simulink model "Missile_Guidance_Solution"  (R2023b)
settings: Solver=ode45  StartTime=0.0  StopTime=20  RelTol=1e-3  AbsTol=1e-6
PreLoadFcn:
  | aero_guid_dat
StopFcn:
  | aero_guid_plot
undefined symbols (not defined in the file or in its folder): Beamwidth, Cm_el, Cm_q, Cz_el, d2r, d_ref, fin_max, fin_min, g, h_ini, K_r, Ks, l_acc, max_acc, max_gimbal, min_gimbal, pos_tgt, S_ref, theta_tgt, Thrust, tors, v_tgt, wgyro, wn_hom, x_ini
libraries: simulink_need_slupdate x11, aerospace x4, aerolibanim x1, simulink x1
CloseFcn:
  | h=findobj('type','figure');if ~isempty(h);close(h);end
Description:
  | Dynamics of a missile engaging a target which is flying straight and level
settings Model: PauseTimes=6  Creator=The MathWorks, Inc.  LastModifiedBy=AmitW
settings SolverCC: AutoScaleAbsTol=off  AlgebraicLoopSolver=TrustRegion
settings DataIOCC: SaveFormat=Array  SaveOutput=off  ReturnWorkspaceOutputs=off  StateSaveName=xbase  OutputSaveName=ybase  SignalLoggingName=sigsOut
settings OptimizationCC: BlockReduction=off  ReuseModelBlockBuffer=off  ExpressionDepthLimit=2147483647  InitFltsAndDblsToZero=on  LifeSpan=inf
settings DebuggingCC: SaveWithParameterizedLinksMsg=none  SignalResolutionControl=TryResolveAllWithWarning  MultiTaskDSMMsg=warning  MultiTaskCondExecSysMsg=none  SigSpecEnsureSampleTimeMsg=none  FcnCallInpInsideContextMsg=warning  UnconnectedInputMsg=warning  UnconnectedOutputMsg=warning  UnconnectedLineMsg=warning  StateNameClashWarn=warning  SFUnexpectedBacktrackingDiag=warning  SFNoUnconditionalDefaultTransitionDiag=warning  SFExecutionAtInitializationDiag=none  ArithmeticOperatorsInVariantConditions=warning
settings HardwareCC: ProdBitPerPointer=32  ProdBitPerSizeT=32  ProdBitPerPtrDiffT=32  ProdLargestAtomicFloat=None  ProdIntDivRoundTo=Undefined  ProdEndianess=Unspecified  ProdWordSize=32  ProdHWDeviceType=32-bit Generic
settings ModelReferenceCC: EnableRefExpFcnMdlSchedulingChecks=on  PropagateSignalLabelsOutOfModel=off
settings SFSimCC: SimUseLocalCustomCode=off  SimParseCustomCode=off  CustomCodeUndefinedFunction=UseInterfaceOnly
settings RTWCC: RTWUseLocalCustomCode=off
settings CodeAppCC: StateflowObjectComments=on
settings GRTTargetCC: TargetFcnLib=ansi_tfl_tmw.mat  TargetLangStandard=C89/C90 (ANSI)  CombineOutputUpdateFcns=off  GRTInterface=on
settings ConfigComp: CovMetricSettings=d  CovSaveCumulativeToWorkspaceVar=on  CovSaveSingleToWorkspaceVar=on  CovExternalEMLEnable=off  CovSFcnEnable=off

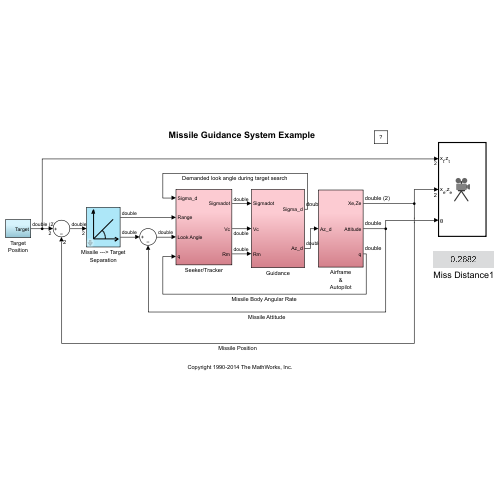
[thumbnail: Simulink's stored preview of the top-level diagram]
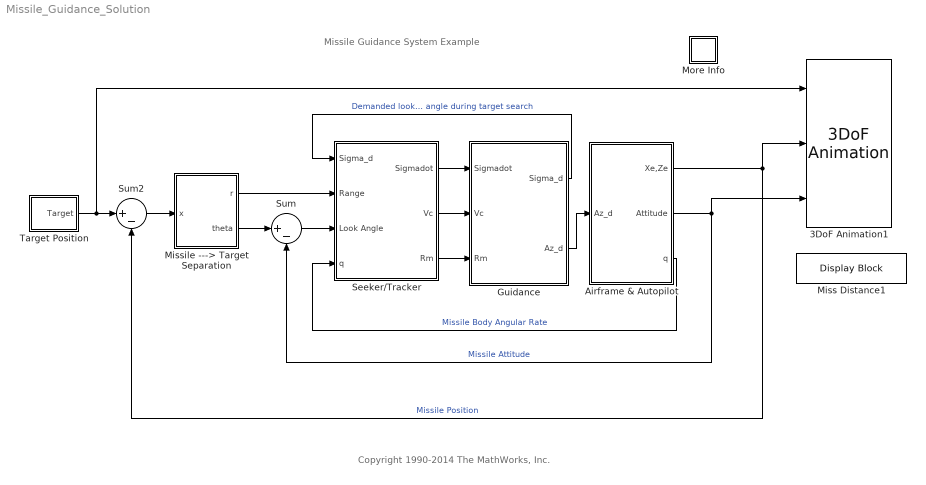
== system Missile_Guidance_Solution ==
  note: Copyright 1990-2014 The MathWorks, Inc.
  note: Missile Guidance System Example
  3DoF Animation1 : aerolibanim/3DoF Animation  u1=[0 5000 -2000 2000 -5050 -3050]  u2=0.01  u3=2.0  u5=Fixed position  u6=[2000 500 -3150]  u7=10  u8=on
  Airframe & Autopilot : Subsystem
  Guidance : Subsystem
  Miss Distance1 : DisplayBlock  LabelPosition=Hide  Transparency=1
  Missile ---> Target Separation : Subsystem  mask(Cart2Polar){}
      mask help:
      | Transformation from cartesian to polar coordinates.
      | [x, y] -> [r, theta]
      |
      | r = sqrt(x^2 + y^2);
      | theta = atan(y/x);
      mask Help: Unmask this block for more help.
      mask Display: plot(0,0,100,100,[24,20,15,20,20],[85,95,85,95,20],[80,20,95,85,95,85],[70,20,20,15,20,24],[56,56,55,52,50,46],[20,26,31,35,38,42])
  More Info : Subsystem
      settings: OpenFcn=showExample('simulink_aerospace/DesigningAGuidanceSystemInMATLABAndSimulinkExample')
      mask Display: disp('?')
  Seeker/Tracker : Subsystem
  Sum : Sum  Inputs=|+-  InputSameDT=on  SaturateOnIntegerOverflow=on  OutDataTypeStr=Inherit: Same as first input
  Sum2 : Sum  Inputs=|+-  InputSameDT=on  SaturateOnIntegerOverflow=on  OutDataTypeStr=Inherit: Same as first input
  Target Position : Subsystem
  wires:
  Missile ---> Target Separation/2(theta) -> Sum/1
  Guidance/2(Az_d) -> Airframe & Autopilot/1(Az_d)
  Seeker/Tracker/2(Vc) -> Guidance/2(Vc)
  Seeker/Tracker/3(Rm) -> Guidance/3(Rm)
  Seeker/Tracker/1(Sigmadot) -> Guidance/1(Sigmadot)
  Sum/1 -> Seeker/Tracker/3(Look Angle)
  Airframe & Autopilot/3(q) -> Seeker/Tracker/4(q)  "Missile Body Angular Rate"
  Guidance/1(Sigma_d) -> Seeker/Tracker/1(Sigma_d)  "Demanded look angle during target search"
  Missile ---> Target Separation/1(r) -> Seeker/Tracker/2(Range)
  Airframe & Autopilot/1(Xe,Ze) -> 3DoF Animation1/2, Sum2/2  "Missile Position"
  Airframe & Autopilot/2(Attitude) -> 3DoF Animation1/3, Sum/2  "Missile Attitude"
  Target Position/1(Target) -> 3DoF Animation1/1, Sum2/1
  Sum2/1 -> Missile ---> Target Separation/1(x)

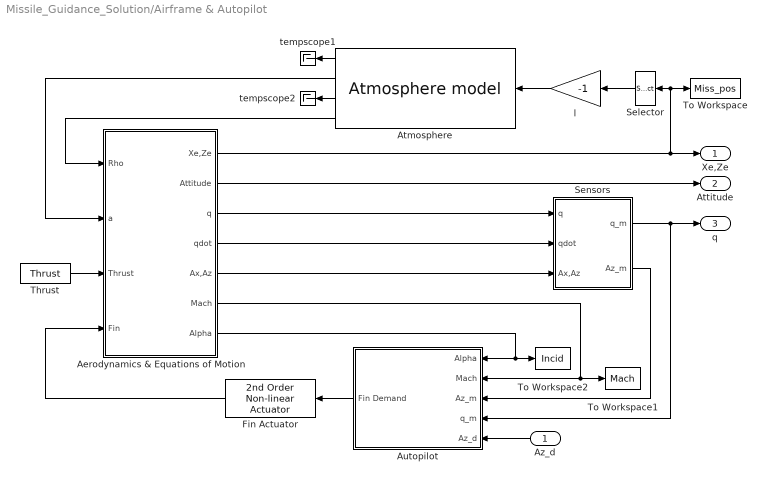
== system Missile_Guidance_Solution/Airframe & Autopilot ==
  Az_d : Inport
  Aerodynamics & Equations of Motion : Subsystem
  Atmosphere : aerospace/Atmosphere/Atmosphere model
  Autopilot : Subsystem
  Fin Actuator : aerospace/Actuators/2nd Order Non-linear Actuator  wn_fin=wn_fin  z_fin=z_fin  fin_max=fin_max  fin_min=fin_min  fin_maxrate=fin_maxrate  fin_act_0=fin_act_0
  Selector : Selector  InputPortWidth=2  IndexOptions=Index vector (dialog)  Indices=[2]  OutputSizes=1
  Sensors : Subsystem
  Thrust : Constant  Value=Thrust
  To Workspace : ToWorkspace  VariableName=Miss_pos  SaveFormat=Structure With Time  SampleTime=-1
  To Workspace1 : ToWorkspace  VariableName=Mach  SaveFormat=Structure With Time  SampleTime=-1
  To Workspace2 : ToWorkspace  VariableName=Incid  SaveFormat=Structure With Time  SampleTime=-1
  l : Gain  Gain=-1  SaturateOnIntegerOverflow=on  OutDataTypeStr=Inherit: Same as input  ParamDataTypeStr=Inherit: Same as input
  tempscope1 : Terminator
  tempscope2 : Terminator
  Xe,Ze : Outport  InitialOutput=0  VectorParamsAs1DForOutWhenUnconnected=off
  Attitude : Outport  Port=2  InitialOutput=0  VectorParamsAs1DForOutWhenUnconnected=off
  q : Outport  Port=3  InitialOutput=0  VectorParamsAs1DForOutWhenUnconnected=off
  wires:
  Aerodynamics & Equations of Motion/2(Attitude) -> Attitude/1
  Thrust/1 -> Aerodynamics & Equations of Motion/3(Thrust)
  Atmosphere/3 -> tempscope2/1
  Atmosphere/4 -> Aerodynamics & Equations of Motion/1(Rho)
  Atmosphere/1 -> tempscope1/1
  Atmosphere/2 -> Aerodynamics & Equations of Motion/2(a)
  Selector/1 -> l/1
  l/1 -> Atmosphere/1
  Aerodynamics & Equations of Motion/5(Ax,Az) -> Sensors/3(Ax,Az)
  Aerodynamics & Equations of Motion/4(qdot) -> Sensors/2(qdot)
  Aerodynamics & Equations of Motion/1(Xe,Ze) -> Xe,Ze/1, To Workspace/1, Selector/1
  Az_d/1 -> Autopilot/5(Az_d)
  Autopilot/1(Fin Demand) -> Fin Actuator/1
  Fin Actuator/1 -> Aerodynamics & Equations of Motion/4(Fin)
  Aerodynamics & Equations of Motion/7(Alpha) -> Autopilot/1(Alpha), To Workspace2/1
  Sensors/2(Az_m) -> Autopilot/3(Az_m)
  Aerodynamics & Equations of Motion/6(Mach) -> Autopilot/2(Mach), To Workspace1/1
  Sensors/1(q_m) -> Autopilot/4(q_m), q/1
  Aerodynamics & Equations of Motion/3(q) -> Sensors/1(q)

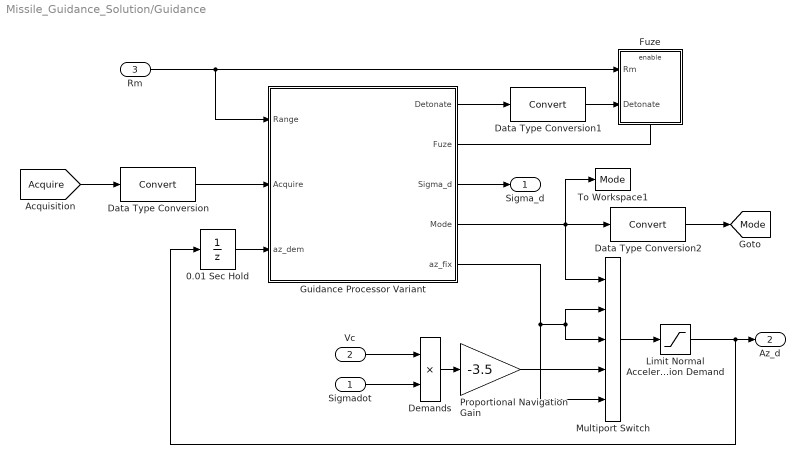
== system Missile_Guidance_Solution/Guidance ==
  Sigmadot : Inport
  Vc : Inport  Port=2
  Rm : Inport  Port=3
  0.01 Sec Hold : UnitDelay  SampleTime=0.01  HasFrameUpgradeWarning=on
  Data Type Conversion : DataTypeConversion  SaturateOnIntegerOverflow=off  RndMeth=Floor
  Data Type Conversion1 : DataTypeConversion  SaturateOnIntegerOverflow=off  RndMeth=Floor
  Data Type Conversion2 : DataTypeConversion  SaturateOnIntegerOverflow=off  RndMeth=Floor
  Demands : Product  InputSameDT=on  SaturateOnIntegerOverflow=on  OutDataTypeStr=Inherit: Same as first input
  Fuze : Subsystem  TreatAsAtomicUnit=on
  Guidance Processor Variant : Subsystem  Variant=on  VariantControlMode=label  LabelModeActiveChoice=Guid_Stateflow  mask(Guidance Processor){VarModel=Stateflow}
      mask prompts: VarModel "Guidance logic implementation"
      mask help:
      | Guidance missile logic.
      | The process works at 100 Hertz.
      mask init:
      | set_param(gcb, 'OverrideUsingVariant', ['Guid_' VarModel]);
      mask TypeOptions VarModel: Matlab | Stateflow
  "Limit Normal Acceleration Demand " : Saturate  UpperLimit=max_acc  LowerLimit=-max_acc
  Multiport Switch : MultiPortSwitch  Inputs=4
  Proportional Navigation Gain : Gain  Gain=-3.5  SaturateOnIntegerOverflow=on  OutDataTypeStr=Inherit: Same as input  ParamDataTypeStr=Inherit: Same as input
  To Workspace1 : ToWorkspace  VariableName=Mode  SaveFormat=Structure With Time
  Sigma_d : Outport  VectorParamsAs1DForOutWhenUnconnected=off
  Az_d : Outport  Port=2  VectorParamsAs1DForOutWhenUnconnected=off
  tag scope: Mode=global
  wires:
  Guidance Processor Variant/3(Sigma_d) -> Sigma_d/1
  [Acquire] -> Data Type Conversion/1
  Multiport Switch/1 -> "Limit Normal Acceleration Demand "/1
  Guidance Processor Variant/1(Detonate) -> Data Type Conversion1/1
  "Limit Normal Acceleration Demand "/1 -> Az_d/1, 0.01 Sec Hold/1
  Guidance Processor Variant/5(az_fix) -> Multiport Switch/2, Multiport Switch/3, Multiport Switch/5
  0.01 Sec Hold/1 -> Guidance Processor Variant/3(az_dem)
  Sigmadot/1 -> Demands/2
  Proportional Navigation Gain/1 -> Multiport Switch/4
  Vc/1 -> Demands/1
  Demands/1 -> Proportional Navigation Gain/1
  Rm/1 -> Guidance Processor Variant/1(Range), Fuze/1(Rm)
  Guidance Processor Variant/2(Fuze) -> Fuze/Enable
  Guidance Processor Variant/4(Mode) -> Data Type Conversion2/1, To Workspace1/1, Multiport Switch/1
  Data Type Conversion/1 -> Guidance Processor Variant/2(Acquire)
  Data Type Conversion1/1 -> Fuze/2(Detonate)
  Data Type Conversion2/1 -> [Mode]

== system Missile_Guidance_Solution/Missile ---> Target Separation ==
  x : Inport
  Range : Fcn  Expr=hypot(u[1],u[2])
  Sightline Angle : Fcn  Expr=atan2(-u[2],u[1])
  r : Outport  InitialOutput=0  VectorParamsAs1DForOutWhenUnconnected=off
  theta : Outport  Port=2  InitialOutput=0  VectorParamsAs1DForOutWhenUnconnected=off
  wires:
  x/1 -> Sightline Angle/1, Range/1
  Range/1 -> r/1
  Sightline Angle/1 -> theta/1

== system Missile_Guidance_Solution/More Info ==

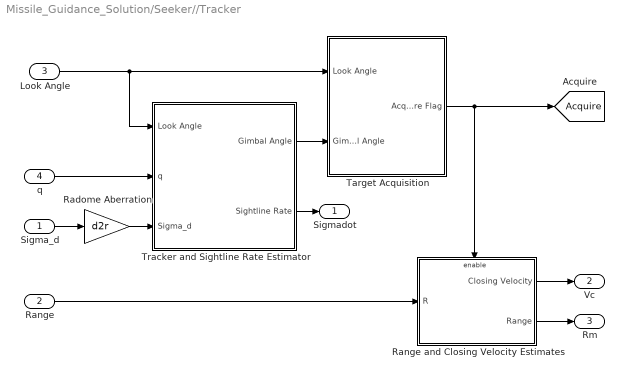
== system Missile_Guidance_Solution/Seeker//Tracker ==
  Sigma_d : Inport
  Range : Inport  Port=2
  Look Angle : Inport  Port=3
  q : Inport  Port=4
  Radome Aberration : Gain  Gain=d2r  SaturateOnIntegerOverflow=on  OutDataTypeStr=Inherit: Same as input  ParamDataTypeStr=Inherit: Same as input
  Range and Closing Velocity Estimates : Subsystem  TreatAsAtomicUnit=on
  Target Acquisition : Subsystem
  Tracker and Sightline Rate Estimator : Subsystem
  Sigmadot : Outport  VectorParamsAs1DForOutWhenUnconnected=off
  Vc : Outport  Port=2  VectorParamsAs1DForOutWhenUnconnected=off
  Rm : Outport  Port=3  VectorParamsAs1DForOutWhenUnconnected=off
  tag scope: Acquire=global
  wires:
  Tracker and Sightline Rate Estimator/2(Sightline Rate) -> Sigmadot/1
  Radome Aberration/1 -> Tracker and Sightline Rate Estimator/3(Sigma_d)
  Tracker and Sightline Rate Estimator/1("Gimbal Angle ") -> Target Acquisition/2(Gimbal Angle)
  Target Acquisition/1(Acquire Flag) -> [Acquire], Range and Closing Velocity Estimates/Enable
  q/1 -> Tracker and Sightline Rate Estimator/2(q)
  Look Angle/1 -> Target Acquisition/1(Look Angle), Tracker and Sightline Rate Estimator/1(Look Angle)
  Range/1 -> Range and Closing Velocity Estimates/1(R)
  Range and Closing Velocity Estimates/2(Range) -> Rm/1
  Range and Closing Velocity Estimates/1(Closing Velocity) -> Vc/1
  Sigma_d/1 -> Radome Aberration/1

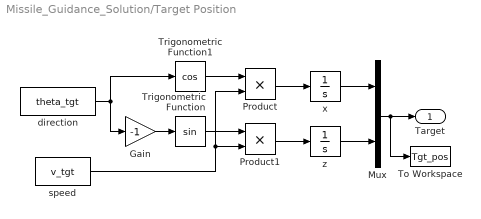
== system Missile_Guidance_Solution/Target Position ==
  Gain : Gain  Gain=-1  SaturateOnIntegerOverflow=on  OutDataTypeStr=Inherit: Same as input  ParamDataTypeStr=Inherit: Same as input
  Mux : Mux  Inputs=2
  Product : Product  InputSameDT=on  SaturateOnIntegerOverflow=on  OutDataTypeStr=Inherit: Same as first input
  Product1 : Product  InputSameDT=on  SaturateOnIntegerOverflow=on  OutDataTypeStr=Inherit: Same as first input
  To Workspace : ToWorkspace  VariableName=Tgt_pos  SaveFormat=Structure  SampleTime=-1
  Trigonometric Function : Trigonometry
  Trigonometric Function1 : Trigonometry  Operator=cos
  direction : Constant  Value=theta_tgt
  speed : Constant  Value=v_tgt
  x : Integrator  InitialCondition=pos_tgt(1)
  z : Integrator  InitialCondition=pos_tgt(2)
  Target : Outport  VectorParamsAs1DForOutWhenUnconnected=off
  wires:
  x/1 -> Mux/1
  z/1 -> Mux/2
  Product/1 -> x/1
  Product1/1 -> z/1
  speed/1 -> Product/2, Product1/2
  Trigonometric Function/1 -> Product1/1
  Trigonometric Function1/1 -> Product/1
  direction/1 -> Trigonometric Function1/1, Gain/1
  Gain/1 -> Trigonometric Function/1
  Mux/1 -> Target/1, To Workspace/1

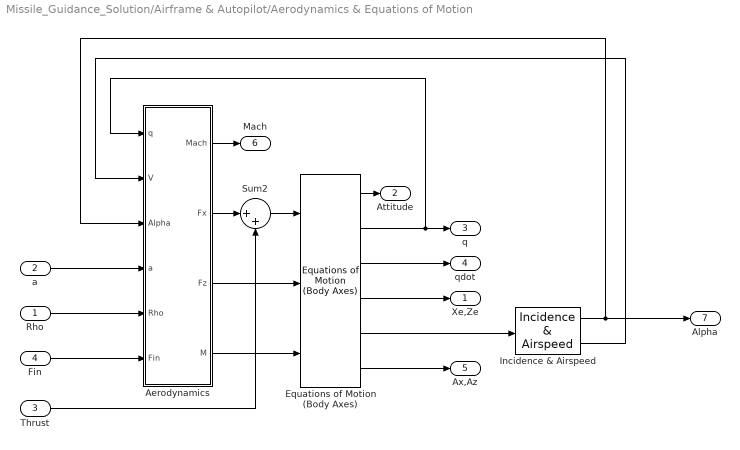
== system Missile_Guidance_Solution/Airframe & Autopilot/Aerodynamics & Equations of Motion ==
  Rho : Inport
  a : Inport  Port=2
  Thrust : Inport  Port=3
  Fin : Inport  Port=4
  " Equations of Motion (Body Axes)" : aerospace/3DoF Equations of Motion / Equations of Motion (Body Axes)  v_ini=v_ini  theta_ini=theta_ini  alpha_ini=alpha_ini  q_ini=q_ini  pos_ini=[x_ini -h_ini]  mass=mass  Iyy=Iyy  g=g
  Aerodynamics : Subsystem
  Incidence & Airspeed : aerospace/3DoF Equations of Motion /Incidence  & Airspeed
  Sum2 : Sum  Inputs=|++  InputSameDT=on  SaturateOnIntegerOverflow=on  OutDataTypeStr=Inherit: Same as first input
  Xe,Ze : Outport  InitialOutput=0  VectorParamsAs1DForOutWhenUnconnected=off
  Attitude : Outport  Port=2  InitialOutput=0  VectorParamsAs1DForOutWhenUnconnected=off
  q : Outport  Port=3  InitialOutput=0  VectorParamsAs1DForOutWhenUnconnected=off
  qdot : Outport  Port=4  InitialOutput=0  VectorParamsAs1DForOutWhenUnconnected=off
  Ax,Az : Outport  Port=5  InitialOutput=0  VectorParamsAs1DForOutWhenUnconnected=off
  Mach : Outport  Port=6  InitialOutput=0  VectorParamsAs1DForOutWhenUnconnected=off
  Alpha : Outport  Port=7  InitialOutput=0  VectorParamsAs1DForOutWhenUnconnected=off
  wires:
  Aerodynamics/1(" Mach") -> Mach/1
  Aerodynamics/4(" M") -> " Equations of Motion (Body Axes)"/3
  Sum2/1 -> " Equations of Motion (Body Axes)"/1
  Incidence & Airspeed/1 -> Aerodynamics/3(Alpha), Alpha/1
  Rho/1 -> Aerodynamics/5(Rho)
  a/1 -> Aerodynamics/4(a)
  Fin/1 -> Aerodynamics/6(Fin)
  Incidence & Airspeed/2 -> Aerodynamics/2(V)
  Aerodynamics/3(Fz) -> " Equations of Motion (Body Axes)"/2
  " Equations of Motion (Body Axes)"/2 -> q/1, Aerodynamics/1(q)
  " Equations of Motion (Body Axes)"/3 -> qdot/1
  " Equations of Motion (Body Axes)"/1 -> Attitude/1
  " Equations of Motion (Body Axes)"/4 -> Xe,Ze/1
  " Equations of Motion (Body Axes)"/6 -> Ax,Az/1
  " Equations of Motion (Body Axes)"/5 -> Incidence & Airspeed/1
  Aerodynamics/2(Fx) -> Sum2/1
  Thrust/1 -> Sum2/2

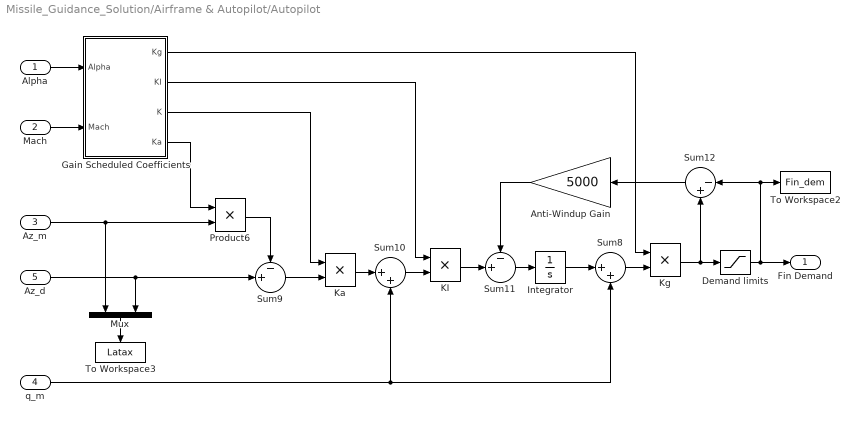
== system Missile_Guidance_Solution/Airframe & Autopilot/Autopilot ==
  Alpha : Inport
  Mach : Inport  Port=2
  Az_m : Inport  Port=3
  q_m : Inport  Port=4
  Az_d : Inport  Port=5
  Anti-Windup Gain : Gain  Gain=5000  SaturateOnIntegerOverflow=on  OutDataTypeStr=Inherit: Same as input  ParamDataTypeStr=Inherit: Same as input
  "Demand limits " : Saturate  UpperLimit=fin_max  LowerLimit=fin_min
  Gain Scheduled Coefficients : Subsystem
  Integrator : Integrator
  KI : Product  InputSameDT=on  SaturateOnIntegerOverflow=on  OutDataTypeStr=Inherit: Same as first input
  Ka : Product  InputSameDT=on  SaturateOnIntegerOverflow=on  OutDataTypeStr=Inherit: Same as first input
  Kg : Product  InputSameDT=on  SaturateOnIntegerOverflow=on  OutDataTypeStr=Inherit: Same as first input
  Mux : Mux  Inputs=2
  Product6 : Product  InputSameDT=on  SaturateOnIntegerOverflow=on  OutDataTypeStr=Inherit: Same as first input
  Sum10 : Sum  Inputs=|++  InputSameDT=on  SaturateOnIntegerOverflow=on  OutDataTypeStr=Inherit: Same as first input
  Sum11 : Sum  Inputs=-+|  InputSameDT=on  SaturateOnIntegerOverflow=on  OutDataTypeStr=Inherit: Same as first input
  Sum12 : Sum  Inputs=|-+  InputSameDT=on  SaturateOnIntegerOverflow=on  OutDataTypeStr=Inherit: Same as first input
  Sum8 : Sum  Inputs=|++  InputSameDT=on  SaturateOnIntegerOverflow=on  OutDataTypeStr=Inherit: Same as first input
  Sum9 : Sum  Inputs=-+|  InputSameDT=on  SaturateOnIntegerOverflow=on  OutDataTypeStr=Inherit: Same as first input
  To Workspace2 : ToWorkspace  VariableName=Fin_dem  SaveFormat=Structure With Time  SampleTime=-1
  To Workspace3 : ToWorkspace  VariableName=Latax  SaveFormat=Structure With Time  SampleTime=-1
  Fin Demand : Outport  InitialOutput=0  VectorParamsAs1DForOutWhenUnconnected=off
  wires:
  Mach/1 -> Gain Scheduled Coefficients/2(Mach)
  Alpha/1 -> Gain Scheduled Coefficients/1(Alpha)
  Kg/1 -> Sum12/2, "Demand limits "/1
  Gain Scheduled Coefficients/1("Kg ") -> Kg/1
  Gain Scheduled Coefficients/3("K ") -> Ka/1
  Gain Scheduled Coefficients/2("KI ") -> KI/1
  Anti-Windup Gain/1 -> Sum11/1
  Sum8/1 -> Kg/2
  Integrator/1 -> Sum8/1
  Sum11/1 -> Integrator/1
  Product6/1 -> Sum9/1
  Sum9/1 -> Ka/2
  Ka/1 -> Sum10/1
  Sum10/1 -> KI/2
  KI/1 -> Sum11/2
  Sum12/1 -> Anti-Windup Gain/1
  Az_d/1 -> Mux/2, Sum9/2
  Mux/1 -> To Workspace3/1
  q_m/1 -> Sum10/2, Sum8/2
  "Demand limits "/1 -> Fin Demand/1, Sum12/1, To Workspace2/1
  Az_m/1 -> Mux/1, Product6/2
  Gain Scheduled Coefficients/4("Ka ") -> Product6/1

== system Missile_Guidance_Solution/Airframe & Autopilot/Sensors ==
  q : Inport
  qdot : Inport  Port=2
  Ax,Az : Inport  Port=3
  Selector : Selector  InputPortWidth=2  IndexOptions=Index vector (dialog)  Indices=[2]  OutputSizes=1
  Sum : Sum  Inputs=-+|  InputSameDT=on  SaturateOnIntegerOverflow=on  OutDataTypeStr=Inherit: Same as first input
  l : Gain  Gain=l_acc  SaturateOnIntegerOverflow=on  OutDataTypeStr=Inherit: Same as input  ParamDataTypeStr=Inherit: Same as input
  q_m : Outport  InitialOutput=0  VectorParamsAs1DForOutWhenUnconnected=off
  Az_m : Outport  Port=2  InitialOutput=0  VectorParamsAs1DForOutWhenUnconnected=off
  wires:
  Selector/1 -> Sum/2
  Ax,Az/1 -> Selector/1
  q/1 -> q_m/1  "Rate Gyro"
  l/1 -> Sum/1
  Sum/1 -> Az_m/1  "Accelerometer"
  qdot/1 -> l/1

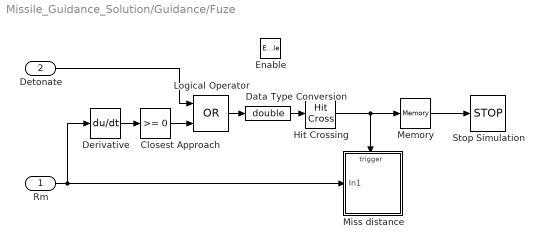
== system Missile_Guidance_Solution/Guidance/Fuze ==
  Rm : Inport
  Detonate : Inport  Port=2
  Enable : EnablePort
  Closest Approach : simulink/Logic and Bit Operations/Compare To Zero  relop=>=  OutDataTypeStr=boolean
  Data Type Conversion : DataTypeConversion  OutDataTypeStr=double  SaturateOnIntegerOverflow=off  RndMeth=Floor
  Derivative : Derivative
  Hit Crossing : HitCross  HitCrossingDirection=rising
  Logical Operator : Logic  Operator=OR  IconShape=distinctive  OutDataTypeStr=boolean
  Memory : Memory
  Miss distance : Subsystem  TreatAsAtomicUnit=on
  Stop Simulation : Stop
  wires:
  Derivative/1 -> Closest Approach/1
  Detonate/1 -> Logical Operator/1
  Rm/1 -> Miss distance/1(In1), Derivative/1
  Closest Approach/1 -> Logical Operator/2
  Memory/1 -> Stop Simulation/1
  Hit Crossing/1 -> Miss distance/Trigger, Memory/1
  Data Type Conversion/1 -> Hit Crossing/1
  Logical Operator/1 -> Data Type Conversion/1

== system Missile_Guidance_Solution/Guidance/Guidance Processor Variant ==
  Range : Inport
  Acquire : Inport  Port=2
  az_dem : Inport  Port=3
  Guidance Processor (MATLAB Function) : Subsystem  TreatAsAtomicUnit=on  PartitionName=GuidaneModel  VariantControl=Guid_Matlab
  Guidance Processor (StateFlow) : Stateflow chart  TreatAsAtomicUnit=on  VariantControl=Guid_Stateflow
  Detonate : Outport
  Fuze : Outport  Port=2
  Sigma_d : Outport  Port=3
  Mode : Outport  Port=4
  az_fix : Outport  Port=5

== system Missile_Guidance_Solution/Seeker//Tracker/Range and Closing Velocity Estimates ==
  R : Inport
  Enable : EnablePort  StatesWhenEnabling=reset
  Bandwidth of Estimator : Gain  Gain=wn_hom  SaturateOnIntegerOverflow=on  OutDataTypeStr=Inherit: Same as input  ParamDataTypeStr=Inherit: Same as input
  Initialized at acquisition : Integrator  InitialConditionSource=external
  Rdot ---> Vc : Gain  Gain=-1  SaturateOnIntegerOverflow=on  OutDataTypeStr=Inherit: Same as input  ParamDataTypeStr=Inherit: Same as input
  Sum : Sum  Inputs=|+-  InputSameDT=on  SaturateOnIntegerOverflow=on  OutDataTypeStr=Inherit: Same as first input
  Closing Velocity : Outport  InitialOutput=0  VectorParamsAs1DForOutWhenUnconnected=off
  Range : Outport  Port=2  InitialOutput=0  VectorParamsAs1DForOutWhenUnconnected=off
  wires:
  R/1 -> Range/1, Initialized at acquisition/2, Sum/1
  Sum/1 -> Bandwidth of Estimator/1
  Initialized at acquisition/1 -> Sum/2
  Bandwidth of Estimator/1 -> Rdot ---> Vc/1, Initialized at acquisition/1
  Rdot ---> Vc/1 -> Closing Velocity/1

== system Missile_Guidance_Solution/Seeker//Tracker/Target Acquisition ==
  Look Angle : Inport
  Gimbal Angle : Inport  Port=2
  Abs : Abs
  Beamwidth : Constant  Value=Beamwidth/2
  Mux : Mux  Inputs=2
  Relational Operator : RelationalOperator  Operator=<  OutDataTypeStr=boolean
  Sum : Sum  Inputs=+-  InputSameDT=on  SaturateOnIntegerOverflow=on  OutDataTypeStr=Inherit: Same as first input
  To Workspace2 : ToWorkspace  VariableName=Gimbal  SaveFormat=Structure With Time  SampleTime=-1
  Acquire Flag : Outport  VectorParamsAs1DForOutWhenUnconnected=off
  wires:
  Look Angle/1 -> Sum/2, Mux/2
  Gimbal Angle/1 -> Sum/1, Mux/1
  Mux/1 -> To Workspace2/1
  Sum/1 -> Abs/1
  Beamwidth/1 -> Relational Operator/2
  Relational Operator/1 -> Acquire Flag/1
  Abs/1 -> Relational Operator/1

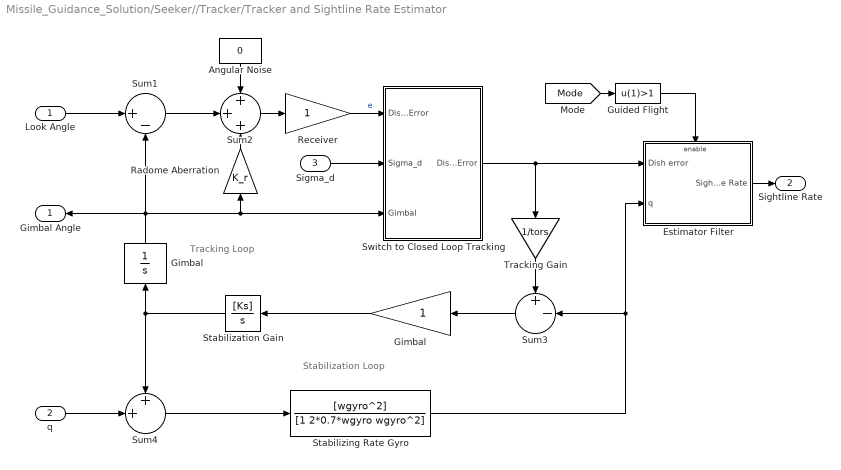
== system Missile_Guidance_Solution/Seeker//Tracker/Tracker and Sightline Rate Estimator ==
  note: Stabilization Loop
  note: Tracking Loop
  Look Angle : Inport
  q : Inport  Port=2
  Sigma_d : Inport  Port=3
  Angular Noise : Constant  Value=0
  Estimator Filter : Subsystem  TreatAsAtomicUnit=on
  Gimbal : Gain  SaturateOnIntegerOverflow=on  OutDataTypeStr=Inherit: Same as input  ParamDataTypeStr=Inherit: Same as input
  "Gimbal " : Integrator  LimitOutput=on  UpperSaturationLimit=max_gimbal  LowerSaturationLimit=min_gimbal
  Guided Flight : Fcn  Expr=u(1)>1
  Radome Aberration : Gain  Gain=K_r  SaturateOnIntegerOverflow=on  OutDataTypeStr=Inherit: Same as input  ParamDataTypeStr=Inherit: Same as input
  Receiver : Gain  SaturateOnIntegerOverflow=on  OutDataTypeStr=Inherit: Same as input  ParamDataTypeStr=Inherit: Same as input
  Stabilization Gain : TransferFcn  Numerator=[Ks]  Denominator=[1 0]
  Stabilizing Rate Gyro : TransferFcn  Numerator=[wgyro^2]  Denominator=[1 2*0.7*wgyro wgyro^2]
  Sum1 : Sum  Inputs=|+-  InputSameDT=on  SaturateOnIntegerOverflow=on  OutDataTypeStr=Inherit: Same as first input
  Sum2 : Sum  Inputs=+++  InputSameDT=on  SaturateOnIntegerOverflow=on  OutDataTypeStr=Inherit: Same as first input
  Sum3 : Sum  Inputs=+-|  InputSameDT=on  SaturateOnIntegerOverflow=on  OutDataTypeStr=Inherit: Same as first input
  Sum4 : Sum  Inputs=++|  InputSameDT=on  SaturateOnIntegerOverflow=on  OutDataTypeStr=Inherit: Same as first input
  Switch to Closed Loop Tracking : Subsystem
  Tracking Gain : Gain  Gain=1/tors  SaturateOnIntegerOverflow=on  OutDataTypeStr=Inherit: Same as input  ParamDataTypeStr=Inherit: Same as input
  "Gimbal Angle " : Outport  VectorParamsAs1DForOutWhenUnconnected=off
  Sightline Rate : Outport  Port=2  VectorParamsAs1DForOutWhenUnconnected=off
  wires:
  "Gimbal "/1 -> Sum1/2, Radome Aberration/1, Switch to Closed Loop Tracking/3(Gimbal), "Gimbal Angle "/1
  Stabilization Gain/1 -> "Gimbal "/1, Sum4/1
  Gimbal/1 -> Stabilization Gain/1
  Look Angle/1 -> Sum1/1
  Sum2/1 -> Receiver/1
  Receiver/1 -> Switch to Closed Loop Tracking/1(Dish Error)  "e"
  Sigma_d/1 -> Switch to Closed Loop Tracking/2(Sigma_d)
  Estimator Filter/1(Sightline Rate) -> Sightline Rate/1
  Radome Aberration/1 -> Sum2/3
  Sum1/1 -> Sum2/2
  Angular Noise/1 -> Sum2/1
  Sum4/1 -> Stabilizing Rate Gyro/1
  q/1 -> Sum4/2
  Stabilizing Rate Gyro/1 -> Sum3/2, Estimator Filter/2(q)
  Sum3/1 -> Gimbal/1
  Tracking Gain/1 -> Sum3/1
  Switch to Closed Loop Tracking/1("Dish Error ") -> Tracking Gain/1, Estimator Filter/1(Dish error)
  Guided Flight/1 -> Estimator Filter/Enable
  [Mode] -> Guided Flight/1

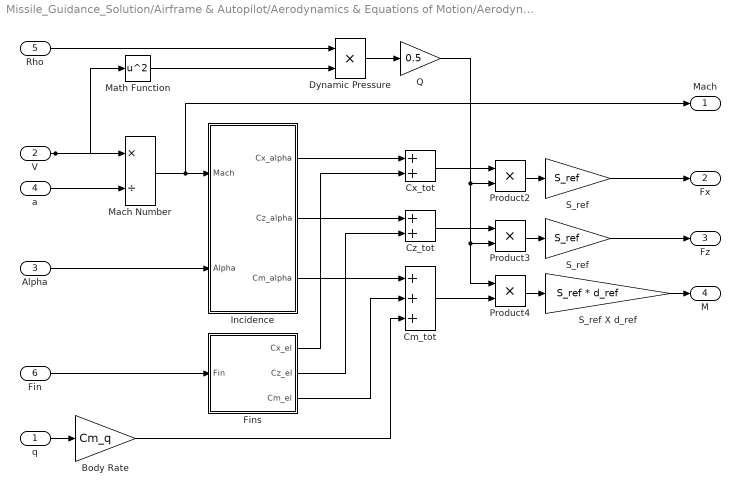
== system Missile_Guidance_Solution/Airframe & Autopilot/Aerodynamics & Equations of Motion/Aerodynamics ==
  q : Inport
  V : Inport  Port=2
  Alpha : Inport  Port=3
  a : Inport  Port=4
  Rho : Inport  Port=5
  Fin : Inport  Port=6
  Body Rate : Gain  Gain=Cm_q  SaturateOnIntegerOverflow=on  OutDataTypeStr=Inherit: Same as input  ParamDataTypeStr=Inherit: Same as input
  Cm_tot : Sum  Inputs=+++  InputSameDT=on  SaturateOnIntegerOverflow=on  OutDataTypeStr=Inherit: Same as first input
  Cx_tot : Sum  InputSameDT=on  SaturateOnIntegerOverflow=on  OutDataTypeStr=Inherit: Same as first input
  Cz_tot : Sum  InputSameDT=on  SaturateOnIntegerOverflow=on  OutDataTypeStr=Inherit: Same as first input
  Dynamic Pressure : Product  InputSameDT=on  SaturateOnIntegerOverflow=on  OutDataTypeStr=Inherit: Same as first input
  Fins : Subsystem
  Incidence : Subsystem
  Mach Number : Product  Inputs=*/  InputSameDT=on  SaturateOnIntegerOverflow=on  OutDataTypeStr=Inherit: Same as first input
  Math Function : Math  Operator=square  SignedPower=on
  Product2 : Product  InputSameDT=on  SaturateOnIntegerOverflow=on  OutDataTypeStr=Inherit: Same as first input
  Product3 : Product  InputSameDT=on  SaturateOnIntegerOverflow=on  OutDataTypeStr=Inherit: Same as first input
  Product4 : Product  InputSameDT=on  SaturateOnIntegerOverflow=on  OutDataTypeStr=Inherit: Same as first input
  Q : Gain  Gain=0.5  SaturateOnIntegerOverflow=on  OutDataTypeStr=Inherit: Same as input  ParamDataTypeStr=Inherit: Same as input
  S_ref : Gain  Gain=S_ref  SaturateOnIntegerOverflow=on  OutDataTypeStr=Inherit: Same as input  ParamDataTypeStr=Inherit: Same as input
  "S_ref " : Gain  Gain=S_ref  SaturateOnIntegerOverflow=on  OutDataTypeStr=Inherit: Same as input  ParamDataTypeStr=Inherit: Same as input
  S_ref X d_ref : Gain  Gain=S_ref * d_ref  SaturateOnIntegerOverflow=on  OutDataTypeStr=Inherit: Same as input  ParamDataTypeStr=Inherit: Same as input
  " Mach" : Outport  InitialOutput=0  VectorParamsAs1DForOutWhenUnconnected=off
  Fx : Outport  Port=2  InitialOutput=[0]  VectorParamsAs1DForOutWhenUnconnected=off
  Fz : Outport  Port=3  InitialOutput=0  VectorParamsAs1DForOutWhenUnconnected=off
  " M" : Outport  Port=4  InitialOutput=0  VectorParamsAs1DForOutWhenUnconnected=off
  wires:
  Math Function/1 -> Dynamic Pressure/2
  Rho/1 -> Dynamic Pressure/1
  Dynamic Pressure/1 -> Q/1
  Q/1 -> Product2/2, Product3/2, Product4/1
  V/1 -> Math Function/1, Mach Number/1
  Incidence/1(Cx_alpha) -> Cx_tot/1
  Fins/1(Cx_el) -> Cx_tot/2
  Incidence/2(Cz_alpha) -> Cz_tot/1
  Fins/2(Cz_el) -> Cz_tot/2
  Incidence/3(Cm_alpha) -> Cm_tot/1
  Fins/3(Cm_el) -> Cm_tot/2
  Body Rate/1 -> Cm_tot/3
  a/1 -> Mach Number/2
  Alpha/1 -> Incidence/2(Alpha)
  Cx_tot/1 -> Product2/1
  Cz_tot/1 -> Product3/1
  Product2/1 -> S_ref/1
  S_ref/1 -> Fx/1
  Product3/1 -> "S_ref "/1
  "S_ref "/1 -> Fz/1
  Fin/1 -> Fins/1(Fin)
  S_ref X d_ref/1 -> " M"/1
  Product4/1 -> S_ref X d_ref/1
  Cm_tot/1 -> Product4/2
  q/1 -> Body Rate/1
  Mach Number/1 -> " Mach"/1, Incidence/1(Mach)

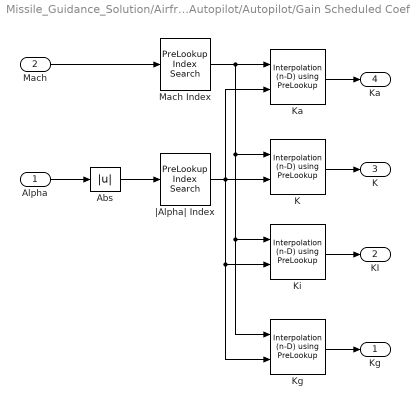
== system Missile_Guidance_Solution/Airframe & Autopilot/Autopilot/Gain Scheduled Coefficients ==
  Alpha : Inport
  Mach : Inport  Port=2
  Abs : Abs
  K : simulink_need_slupdate/Interpolation (n-D) using PreLookup  numDimsPopupSelect=2  explicitNumDims=2  table=K  interpMethod=Linear  extrapMethod=Linear  rangeErrorMode=None  NumSelectionDims=0
  Ka : simulink_need_slupdate/Interpolation (n-D) using PreLookup  numDimsPopupSelect=2  explicitNumDims=2  table=Ka  interpMethod=Linear  extrapMethod=Linear  rangeErrorMode=None  NumSelectionDims=0
  Kg : simulink_need_slupdate/Interpolation (n-D) using PreLookup  numDimsPopupSelect=2  explicitNumDims=2  table=Kg  interpMethod=Linear  extrapMethod=Linear  rangeErrorMode=None  NumSelectionDims=0
  Ki : simulink_need_slupdate/Interpolation (n-D) using PreLookup  numDimsPopupSelect=2  explicitNumDims=2  table=Ki  interpMethod=Linear  extrapMethod=Linear  rangeErrorMode=None  NumSelectionDims=0
  Mach Index : simulink_need_slupdate/PreLookup Index Search  bpData=M_sch  searchMode=Binary Search  cacheBpFlag=on  outputFlag=off  IndexDataType=uint32  extrapMode=Linear Extrapolation  rangeErrorMode=None
  |Alpha| Index : simulink_need_slupdate/PreLookup Index Search  bpData=alpha_sch  searchMode=Binary Search  cacheBpFlag=on  outputFlag=off  IndexDataType=uint32  extrapMode=Linear Extrapolation  rangeErrorMode=None
  "Kg " : Outport  InitialOutput=0  VectorParamsAs1DForOutWhenUnconnected=off
  "KI " : Outport  Port=2  InitialOutput=0  VectorParamsAs1DForOutWhenUnconnected=off
  "K " : Outport  Port=3  InitialOutput=0  VectorParamsAs1DForOutWhenUnconnected=off
  "Ka " : Outport  Port=4  InitialOutput=0  VectorParamsAs1DForOutWhenUnconnected=off
  wires:
  Alpha/1 -> Abs/1
  Mach Index/1 -> Ka/1, K/1, Ki/1, Kg/1
  |Alpha| Index/1 -> Ka/2, K/2, Ki/2, Kg/2
  Ka/1 -> "Ka "/1
  K/1 -> "K "/1
  Ki/1 -> "KI "/1
  Kg/1 -> "Kg "/1
  Abs/1 -> |Alpha| Index/1
  Mach/1 -> Mach Index/1

== system Missile_Guidance_Solution/Guidance/Fuze/Miss distance ==
  In1 : Inport
  Trigger : TriggerPort  VariantControl=(inherit)
  Display : Display
  wires:
  In1/1 -> Display/1

== system Missile_Guidance_Solution/Guidance/Guidance Processor Variant/Guidance Processor (MATLAB Function) ==
  Range : Inport  SampleTime=0.01
  Acquire : Inport  Port=2  SampleTime=0.01
  az_dem : Inport  Port=3  SampleTime=0.01
  Digital Clock : DigitalClock  SampleTime=0.01
  Inner Guidance Processor (MATLAB Function) : MATLAB Function  TreatAsAtomicUnit=on
  Detonate : Outport
  Fuze : Outport  Port=2
  Sigma_d : Outport  Port=3
  Mode : Outport  Port=4
  az_fix : Outport  Port=5
  wires:
  Inner Guidance Processor (MATLAB Function)/1(Detonate) -> Detonate/1
  Digital Clock/1 -> Inner Guidance Processor (MATLAB Function)/4(clock)
  Range/1 -> Inner Guidance Processor (MATLAB Function)/1(Range)
  az_dem/1 -> Inner Guidance Processor (MATLAB Function)/3(az_dem)
  Inner Guidance Processor (MATLAB Function)/5(az_fix) -> az_fix/1
  Inner Guidance Processor (MATLAB Function)/4(Mode) -> Mode/1
  Inner Guidance Processor (MATLAB Function)/3(Sigma_d) -> Sigma_d/1
  Inner Guidance Processor (MATLAB Function)/2(Fuze) -> Fuze/1
  Acquire/1 -> Inner Guidance Processor (MATLAB Function)/2(Acquire)

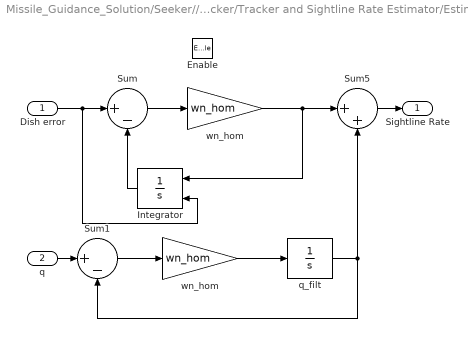
== system Missile_Guidance_Solution/Seeker//Tracker/Tracker and Sightline Rate Estimator/Estimator Filter ==
  Dish error : Inport
  q : Inport  Port=2
  Enable : EnablePort  StatesWhenEnabling=reset
  Integrator : Integrator  InitialConditionSource=external
  Sum : Sum  Inputs=|+-  InputSameDT=on  SaturateOnIntegerOverflow=on  OutDataTypeStr=Inherit: Same as first input
  Sum1 : Sum  Inputs=|+-  InputSameDT=on  SaturateOnIntegerOverflow=on  OutDataTypeStr=Inherit: Same as first input
  Sum5 : Sum  Inputs=|++  InputSameDT=on  SaturateOnIntegerOverflow=on  OutDataTypeStr=Inherit: Same as first input
  q_filt : Integrator
  wn_hom : Gain  Gain=wn_hom  SaturateOnIntegerOverflow=on  OutDataTypeStr=Inherit: Same as input  ParamDataTypeStr=Inherit: Same as input
  "wn_hom  " : Gain  Gain=wn_hom  SaturateOnIntegerOverflow=on  OutDataTypeStr=Inherit: Same as input  ParamDataTypeStr=Inherit: Same as input
  Sightline Rate : Outport  InitialOutput=0  VectorParamsAs1DForOutWhenUnconnected=off
  wires:
  Dish error/1 -> Sum/1, Integrator/2
  Sum/1 -> wn_hom/1
  Integrator/1 -> Sum/2
  Sum5/1 -> Sightline Rate/1
  wn_hom/1 -> Integrator/1, Sum5/1
  q/1 -> Sum1/1
  Sum1/1 -> "wn_hom  "/1
  "wn_hom  "/1 -> q_filt/1
  q_filt/1 -> Sum5/2, Sum1/2

== system Missile_Guidance_Solution/Seeker//Tracker/Tracker and Sightline Rate Estimator/Switch to Closed Loop Tracking ==
  Dish Error : Inport
  Sigma_d : Inport  Port=2
  Gimbal : Inport  Port=3
  Guided Flight : Fcn  Expr=u(1)>1
  Sum5 : Sum  Inputs=-+  InputSameDT=on  SaturateOnIntegerOverflow=on  OutDataTypeStr=Inherit: Same as first input
  Switch2 : Switch  Threshold=0.5
  "Dish Error " : Outport  VectorParamsAs1DForOutWhenUnconnected=off
  wires:
  [Mode] -> Guided Flight/1
  Guided Flight/1 -> Switch2/2
  Sum5/1 -> Switch2/3
  Dish Error/1 -> Switch2/1
  Switch2/1 -> "Dish Error "/1
  Sigma_d/1 -> Sum5/2
  Gimbal/1 -> Sum5/1

== system Missile_Guidance_Solution/Airframe & Autopilot/Aerodynamics & Equations of Motion/Aerodynamics/Fins ==
  Fin : Inport
  Cm : Gain  Gain=Cm_el  SaturateOnIntegerOverflow=on  OutDataTypeStr=Inherit: Same as input  ParamDataTypeStr=Inherit: Same as input
  Cx : Gain  Gain=0  SaturateOnIntegerOverflow=on  OutDataTypeStr=Inherit: Same as input  ParamDataTypeStr=Inherit: Same as input
  Cz : Gain  Gain=Cz_el  SaturateOnIntegerOverflow=on  OutDataTypeStr=Inherit: Same as input  ParamDataTypeStr=Inherit: Same as input
  Cx_el : Outport  InitialOutput=0  VectorParamsAs1DForOutWhenUnconnected=off
  Cz_el : Outport  Port=2  InitialOutput=0  VectorParamsAs1DForOutWhenUnconnected=off
  Cm_el : Outport  Port=3  InitialOutput=0  VectorParamsAs1DForOutWhenUnconnected=off
  wires:
  Fin/1 -> Cx/1, Cm/1, Cz/1
  Cx/1 -> Cx_el/1
  Cm/1 -> Cm_el/1
  Cz/1 -> Cz_el/1

== system Missile_Guidance_Solution/Airframe & Autopilot/Aerodynamics & Equations of Motion/Aerodynamics/Incidence ==
  Mach : Inport
  Alpha : Inport  Port=2
  Alpha Index : simulink_need_slupdate/PreLookup Index Search  bpData=alpha_vec  searchMode=Binary Search  cacheBpFlag=on  outputFlag=off  IndexDataType=uint32  extrapMode=Linear Extrapolation  rangeErrorMode=None
  Cm : simulink_need_slupdate/Interpolation (n-D) using PreLookup  numDimsPopupSelect=2  explicitNumDims=2  table=Cm_alpha  interpMethod=Linear  extrapMethod=Linear  rangeErrorMode=None  NumSelectionDims=0
  Cx : simulink_need_slupdate/Interpolation (n-D) using PreLookup  numDimsPopupSelect=2  explicitNumDims=2  table=Cx_alpha  interpMethod=Linear  extrapMethod=Linear  rangeErrorMode=None  NumSelectionDims=0
  Cz : simulink_need_slupdate/Interpolation (n-D) using PreLookup  numDimsPopupSelect=2  explicitNumDims=2  table=Cz_alpha  interpMethod=Linear  extrapMethod=Linear  rangeErrorMode=None  NumSelectionDims=0
  Mach Index : simulink_need_slupdate/PreLookup Index Search  bpData=Mach_vec  searchMode=Binary Search  cacheBpFlag=on  outputFlag=off  IndexDataType=uint32  extrapMode=Linear Extrapolation  rangeErrorMode=None
  Cx_alpha : Outport  InitialOutput=0  VectorParamsAs1DForOutWhenUnconnected=off
  Cz_alpha : Outport  Port=2  InitialOutput=0  VectorParamsAs1DForOutWhenUnconnected=off
  Cm_alpha : Outport  Port=3  InitialOutput=0  VectorParamsAs1DForOutWhenUnconnected=off
  wires:
  Alpha Index/1 -> Cx/1, Cz/1, Cm/1
  Mach Index/1 -> Cx/2, Cz/2, Cm/2
  Cx/1 -> Cx_alpha/1
  Cz/1 -> Cz_alpha/1
  Cm/1 -> Cm_alpha/1
  Alpha/1 -> Alpha Index/1
  Mach/1 -> Mach Index/1

== matlab function Missile_Guidance_Solution/Guidance/Guidance Processor Variant/Guidance Processor (MATLAB Function)/Inner Guidance Processor (MATLAB Function) ==
  data: Range input; Detonate output; Acquire input; az_dem input; clock input; Fuze output; Sigma_d output; Mode output; az_fix output
function [Detonate, Fuze, Sigma_d, Mode, az_fix] = GuidanceFuzeLogic(Range, Acquire, az_dem, clock)
% Guidance and Fuze logic
persistent Acquire_time     % [sec] Timestamp for acquiring target
persistent sigma_in         % [deg] Demanded look angle for the target
persistent incr             % [deg] increment of the demanded look angle for the target
persistent guidMod_in       % [enum] Guidance states 
persistent fuzeMod_in       % [enum] Fuze states
persistent az_fix_in        % [rad] fixed azimuth command

if isempty(Acquire_time);   Acquire_time = clock;   end
if isempty(sigma_in);       sigma_in     = 0;       end
if isempty(az_fix_in);      az_fix_in    = 0;       end
if isempty(incr);           incr         = 0;       end
if isempty(guidMod_in);     guidMod_in   = 0;       end
if isempty(fuzeMod_in);     fuzeMod_in   = 0;       end

Timeout     = false;        % [bool] Acquisition timeout flag
Detonate    = 0;
Fuze        = 0;

 
%% Guidance

switch guidMod_in
    case 0                                  % Init         
        guidMod_in      = 1;
        Acquire_time    = clock;
        incr            = -100;
        sigma_in        = 0;        
        az_fix_in       = -9.81;
    
    case 1                                  % Target Search
        % State transition condition
        if Acquire == 1
            guidMod_in   = 2;
            Acquire_time = clock;
        elseif clock - Acquire_time > 7
            guidMod_in   = 5;
            Timeout      = true;
            Detonate     = 1;
        else
            sigma_in     = sigma_in + 0.01*incr;     
        
            % Inner state condition
            if sigma_in > 30 || sigma_in < -30
                incr     = -incr;                % Write here error
            end 
        end        
           
    case 2                                  % Target Lock
        % State transition condition
        if clock - Acquire_time > 0.2           % Write here error
            guidMod_in = 3;
        end
            
    case 3                                  % Radar Guided     
        % State transition condition
        if Acquire == 0
            guidMod_in   = 1;
            Acquire_time = clock;
            incr         = -100;
            sigma_in     = 0;
        elseif Range < 200
            az_fix_in    = az_dem;
            guidMod_in   = 4;            
        end

    case 4                                  % Blind Range
        % Endgame - Do nothing

    case 5                                  % Abort
        Detonate     = 1;
end


%% Fuze

switch fuzeMod_in
    case 0                                  % Init / Inert
        Fuze = 0;
        
        % State transition condition
        if Timeout || ...
            (guidMod_in == 3 && Range < 1000)
            fuzeMod_in  = 1;
            Fuze        = 1;
        end

    case 1                                  % Armed    
        Fuze = 1;

        % State transition condition
        if guidMod_in == 1
            Fuze        = 0;
            fuzeMod_in  = 0;            
        end
end


%% Finish

Mode    = guidMod_in;
Sigma_d = sigma_in;
az_fix  = az_fix_in;

end

== stateflow chart Missile_Guidance_Solution/Guidance/Guidance Processor Variant/Guidance Processor (StateFlow) ==
  settings: updateMethod=DISCRETE  sampleTime=0.01
  state Guidance [parallel]
    settings: executionOrder=1
    state Target_Search
      en: Mode=1;Sigma_d=0;incr=-100;Acquire_time=t;
      du: Sigma_d=Sigma_d+0.01*incr;
      Target_Search -> Target_Search [order 1] : [Sigma_d>30||Sigma_d<-30]  / incr=-incr;
    state Target_Lock
      en:Mode=2;Acquire_time=t;
    state Abort
      en:Detonate=1;
    state Radar_Guided
      en:Mode=3;
      ex:az_fix=az_dem;
    state Blind_Range
      en:Mode=4;
    (default) -> Target_Search : {az_fix=-9.81;}
    Radar_Guided -> Target_Search [order 1] : [Acquire==0]
    Target_Search -> Abort [order 2] : [t-Acquire_time>7]
        | / send(Timeout, Fuze);
    Target_Search -> Target_Lock [order 1] : [Acquire==1]
    Target_Lock -> Radar_Guided : [t-Acquire_time>0.2]
    Radar_Guided -> Blind_Range [order 2] : [Range<200]
  state Fuze [parallel]
    settings: executionOrder=2
    state Armed
      en:Fuze=1;
    state Inert
      en:Fuze = 0;
    Inert -> Armed [order 2] : [in(Guidance.Radar_Guided)&&Range<1000]
    (default) -> Inert
    Inert -> Armed [order 1] : Timeout
    Armed -> Inert : enter(Guidance.Target_Search)
  data: Range input double [0..]; Detonate output boolean; Fuze output boolean; Sigma_d output double; Mode output uint8; Acquire input boolean; Acquire_time local double; incr local double; az_dem input double; az_fix output double =-9.81
  data Sigma_d settings: description=Demanded Seeker Look Angle
  data Acquire settings: description=Seeker Acquisition Flag
  data incr settings: description=Seeker Search Rate
  events: Timeout local EITHER_EDGE_EVENT
